simulink library "Lab_Library"  (R2022b)
settings: Solver=VariableStepAuto  StartTime=0.0  StopTime=10.0  RelTol=1e-3
undefined symbols (not defined in the file): IO397
libraries: slrealtimeiplib x7, slrealtimeseriallib x1, speedgoatlib_fpga_spi x1, speedgoatlib_fpga x1
settings Model: Creator=l-zirwin  LastModifiedBy=l-zirwin

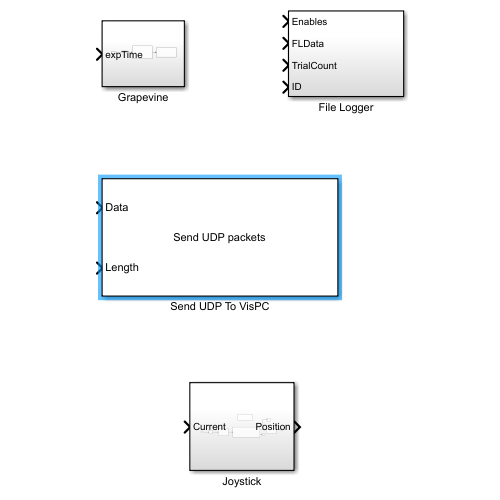
[thumbnail: Simulink's stored preview of the top-level diagram]
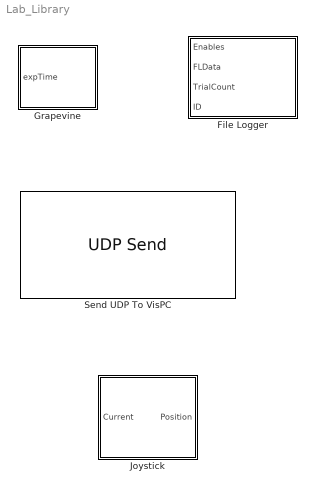
== system Lab_Library ==
  File Logger : Subsystem
  Grapevine : Subsystem
  Joystick : Subsystem
  Send UDP To VisPC : slrealtimeiplib/UDP Send  useHostTargetConn=off  toAddress='192.168.44.2'  toPort=11114  sampleTime=-1  enableMessage=off  ipAddress='192.168.44.1'  localPort=11114

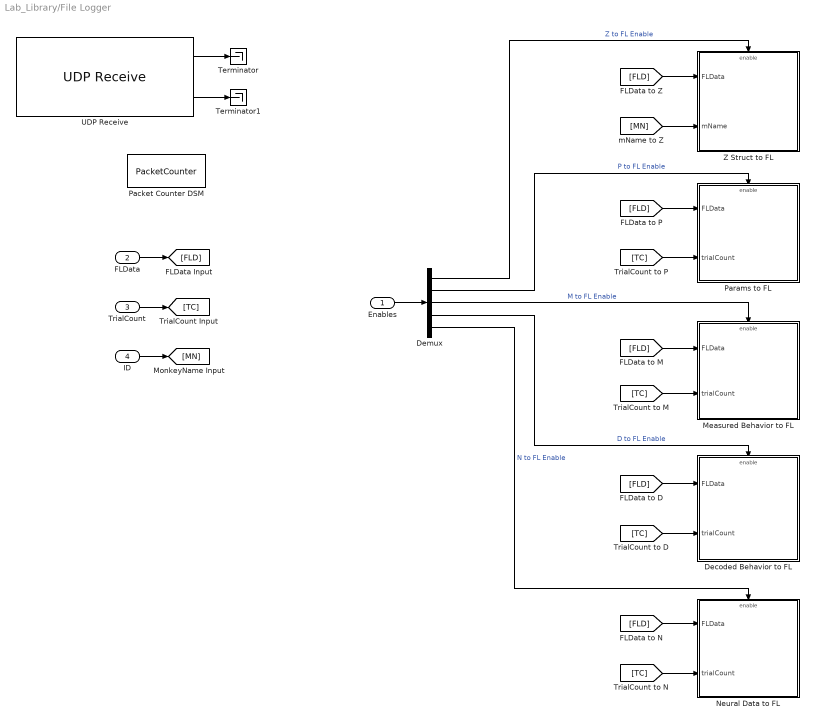
== system Lab_Library/File Logger ==
  Enables : Inport  OutDataTypeStr=uint8  PortDimensions=[1 5]
  FLData : Inport  Port=2  OutDataTypeStr=Bus: FileLoggerEntry
  TrialCount : Inport  Port=3
  ID : Inport  Port=4
  Decoded Behavior to FL : Subsystem
  Demux : Demux  Outputs=5
  Measured Behavior to FL : Subsystem
  Neural Data to FL : Subsystem
  Packet Counter DSM : DataStoreMemory  DataStoreName=PacketCounter  WriteAfterWriteMsg=warning  ShowAdditionalParam=off  OutDataTypeStr=uint32  Dimensions=1
  Params to FL : Subsystem
  Terminator : Terminator
  Terminator1 : Terminator
  UDP Receive : slrealtimeiplib/UDP Receive  useHostTargetConn=off  ipAddress='192.168.43.1'  localPort=11114  rcvWidth=16  rcvFmAny=off  fmAddress='192.168.43.2'  sampleTime=-1  enableMessage=off  maxPackets=1
  Z Struct to FL : Subsystem
  wires:
  TrialCount/1 -> [TC]
  FLData/1 -> [FLD]
  [FLD] -> Z Struct to FL/1(FLData)
  [FLD] -> Params to FL/1(FLData)
  [FLD] -> Measured Behavior to FL/1(FLData)
  [FLD] -> Decoded Behavior to FL/1(FLData)
  [FLD] -> Neural Data to FL/1(FLData)
  [TC] -> Params to FL/2(trialCount)
  [TC] -> Measured Behavior to FL/2(trialCount)
  [TC] -> Decoded Behavior to FL/2(trialCount)
  [TC] -> Neural Data to FL/2(trialCount)
  Enables/1 -> Demux/1
  Demux/3 -> Measured Behavior to FL/Enable  "M to FL Enable"
  Demux/4 -> Decoded Behavior to FL/Enable  "D to FL Enable"
  Demux/5 -> Neural Data to FL/Enable  "N to FL Enable"
  Demux/2 -> Params to FL/Enable  "P to FL Enable"
  Demux/1 -> Z Struct to FL/Enable  "Z to FL Enable"
  ID/1 -> [MN]
  [MN] -> Z Struct to FL/2(mName)
  UDP Receive/2 -> Terminator1/1
  UDP Receive/1 -> Terminator/1

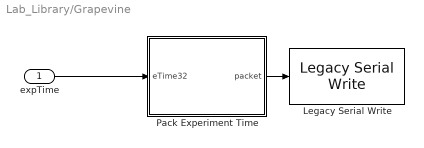
== system Lab_Library/Grapevine ==
  expTime : Inport
  Legacy Serial Write : slrealtimeseriallib/Mainboard/Legacy Serial Write  port=Legacy Serial Port 2  dtype=count+32 bit uint  sampletime=-1
  Pack Experiment Time : MATLAB Function  TreatAsAtomicUnit=on
  wires:
  expTime/1 -> Pack Experiment Time/1(eTime32)
  Pack Experiment Time/1(packet) -> Legacy Serial Write/1

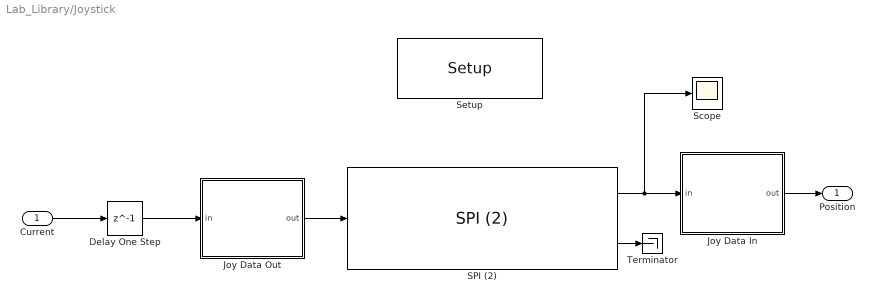
== system Lab_Library/Joystick ==
  Current : Inport
  Delay One Step : Delay  DelayLength=1
  Joy Data In : MATLAB Function  TreatAsAtomicUnit=on
  Joy Data Out : MATLAB Function  TreatAsAtomicUnit=on
  SPI (2) : speedgoatlib_fpga_spi/SPI (2)  id=1  chan=[1]  samp_time=.001  board=IO397-50k  pciSlot=-1  role=Master  sync_mode=off  multislave_mode=off  write_only=off  read_only=off  enableDma=off  multislave_chan=[1]  cpol=[0]  cpha=[0]  frequency=[1e6]  frequency_eff=1e6  delay_start=[2e-6]  delay_start_eff=2e-6  delay_interword=[1e-6]  delay_interword_eff=1e-6  delay_stop=[1e-6]  delay_stop_eff=1e-6  delay_compensation=[100e-9]  delay_compensation_eff=106.7e-9  words_per_frame=[2]  dynamic_words_per_frame=off  bits_per_word=[16]  bit_shift_lsb_first=[0]  no_cs=off  clock_timeout=[1e-6]  clock_timeout_eff=1E-06
      settings: SourceProductName=Simulink Real-Time: Speedgoat I/O Blockset
  Scope : Scope
  Setup : speedgoatlib_fpga/Setup/Setup  board=IO397-50k  id=1  device_id=1  frontIO=None  rearIO=None  bitstreamFile=speedgoat_IO397_50k_Comms.mat  rev=4.000000  timestamp_string=18/02/22 13:58:38  fpgaFreq=75 MHz  fpgaTick=13.33 ns  ProgSpiFlash=off  ProgBPIFlash=off  pciSlot=-1  PullRPort0=pull-up 3.3V  VioPort0=3.3V  PullRPort1=pull-up 3.3V  VioPort1=3.3V  PullRPort2=pull-up 3.3V  VioPort2=3.3V  PullRPort3=pull-up 3.3V  VioPort3=3.3V  PullRPort4=pull-up 3.3V  VioPort4=3.3V  PullRPort5=pull-up 3.3V  VioPort5=3.3V  PullRPort6=pull-up 3.3V  VioPort6=3.3V  diffLineTermination_rear1=on  diffLineTermination_rear2=on  diffLineTermination_rear3=on  diffLineTermination_rear4=on  diffLineTermination_rear5=on  diffLineTermination_rear6=on  diffLineTermination_rear7=on  diffLineTermination_rear8=on  PullRPort15=pull-up 3.3V  PullRPort31=pull-up 3.3V  PullRPort47=pull-up 3.3V  PullRPort63=pull-up 3.3V  diffLineTermination_1=on  diffLineTermination_2=on  diffLineTermination_3=on  diffLineTermination_4=on  diffLineTermination_5=on  diffLineTermination_6=on  diffLineTermination_7=on  diffLineTermination_8=on
      settings: SourceProductName=Simulink Real-Time: Speedgoat I/O Blockset
  Terminator : Terminator
  Position : Outport
  wires:
  Joy Data Out/1(out) -> SPI (2)/1
  SPI (2)/1 -> Scope/1, Joy Data In/1(in)
  Joy Data In/1(out) -> Position/1
  SPI (2)/2 -> Terminator/1
  Current/1 -> Delay One Step/1
  Delay One Step/1 -> Joy Data Out/1(in)

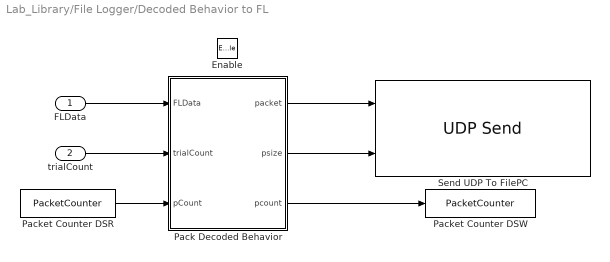
== system Lab_Library/File Logger/Decoded Behavior to FL ==
  FLData : Inport
  trialCount : Inport  Port=2
  Enable : EnablePort
  Pack Decoded Behavior : MATLAB Function  TreatAsAtomicUnit=on
  Packet Counter DSR : DataStoreRead  DataStoreName=PacketCounter  SampleTime=.001  IndexOptions=Index vector (dialog)  Indices=1  OutputSizes=1
  Packet Counter DSW : DataStoreWrite  DataStoreName=PacketCounter  IndexOptions=Index vector (dialog)  Indices=1  OutputSizes=1
  Send UDP To FilePC : slrealtimeiplib/UDP Send  useHostTargetConn=off  toAddress='192.168.43.2'  toPort=11114  sampleTime=-1  enableMessage=off  ipAddress='192.168.43.1'  localPort=11114
  wires:
  FLData/1 -> Pack Decoded Behavior/1(FLData)
  trialCount/1 -> Pack Decoded Behavior/2(trialCount)
  Packet Counter DSR/1 -> Pack Decoded Behavior/3(pCount)
  Pack Decoded Behavior/1(packet) -> Send UDP To FilePC/1
  Pack Decoded Behavior/3(pcount) -> Packet Counter DSW/1
  Pack Decoded Behavior/2(psize) -> Send UDP To FilePC/2

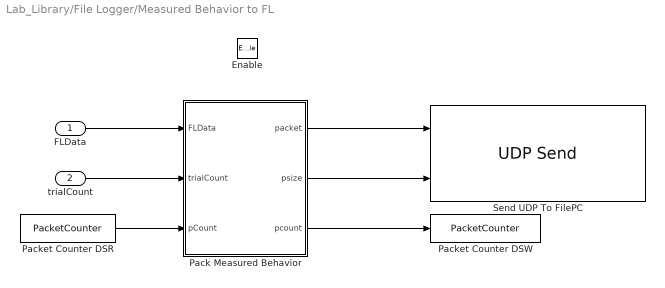
== system Lab_Library/File Logger/Measured Behavior to FL ==
  FLData : Inport
  trialCount : Inport  Port=2
  Enable : EnablePort
  Pack Measured Behavior : MATLAB Function  TreatAsAtomicUnit=on
  Packet Counter DSR : DataStoreRead  DataStoreName=PacketCounter  SampleTime=.001  IndexOptions=Index vector (dialog)  Indices=1  OutputSizes=1
  Packet Counter DSW : DataStoreWrite  DataStoreName=PacketCounter  IndexOptions=Index vector (dialog)  Indices=1  OutputSizes=1
  Send UDP To FilePC : slrealtimeiplib/UDP Send  useHostTargetConn=off  toAddress='192.168.43.2'  toPort=11114  sampleTime=-1  enableMessage=off  ipAddress='192.168.43.1'  localPort=11114
  wires:
  FLData/1 -> Pack Measured Behavior/1(FLData)
  trialCount/1 -> Pack Measured Behavior/2(trialCount)
  Packet Counter DSR/1 -> Pack Measured Behavior/3(pCount)
  Pack Measured Behavior/3(pcount) -> Packet Counter DSW/1
  Pack Measured Behavior/1(packet) -> Send UDP To FilePC/1
  Pack Measured Behavior/2(psize) -> Send UDP To FilePC/2

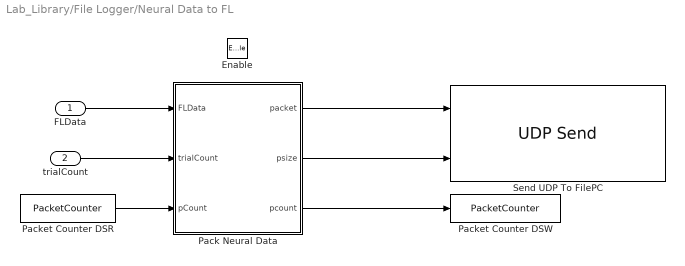
== system Lab_Library/File Logger/Neural Data to FL ==
  FLData : Inport
  trialCount : Inport  Port=2
  Enable : EnablePort
  Pack Neural Data : MATLAB Function  TreatAsAtomicUnit=on
  Packet Counter DSR : DataStoreRead  DataStoreName=PacketCounter  SampleTime=.001  IndexOptions=Index vector (dialog)  Indices=1  OutputSizes=1
  Packet Counter DSW : DataStoreWrite  DataStoreName=PacketCounter  IndexOptions=Index vector (dialog)  Indices=1  OutputSizes=1
  Send UDP To FilePC : slrealtimeiplib/UDP Send  useHostTargetConn=off  toAddress='192.168.43.2'  toPort=11114  sampleTime=-1  enableMessage=off  ipAddress='192.168.43.1'  localPort=11114
  wires:
  FLData/1 -> Pack Neural Data/1(FLData)
  trialCount/1 -> Pack Neural Data/2(trialCount)
  Packet Counter DSR/1 -> Pack Neural Data/3(pCount)
  Pack Neural Data/3(pcount) -> Packet Counter DSW/1
  Pack Neural Data/1(packet) -> Send UDP To FilePC/1
  Pack Neural Data/2(psize) -> Send UDP To FilePC/2

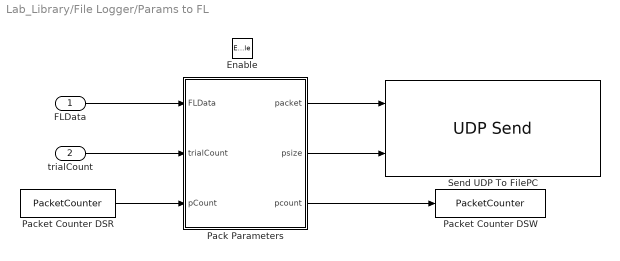
== system Lab_Library/File Logger/Params to FL ==
  FLData : Inport
  trialCount : Inport  Port=2
  Enable : EnablePort
  Pack Parameters : MATLAB Function  TreatAsAtomicUnit=on
  Packet Counter DSR : DataStoreRead  DataStoreName=PacketCounter  SampleTime=.001  IndexOptions=Index vector (dialog)  Indices=1  OutputSizes=1
  Packet Counter DSW : DataStoreWrite  DataStoreName=PacketCounter  IndexOptions=Index vector (dialog)  Indices=1  OutputSizes=1
  Send UDP To FilePC : slrealtimeiplib/UDP Send  useHostTargetConn=off  toAddress='192.168.43.2'  toPort=11114  sampleTime=-1  enableMessage=off  ipAddress='192.168.43.1'  localPort=11114
  wires:
  FLData/1 -> Pack Parameters/1(FLData)
  trialCount/1 -> Pack Parameters/2(trialCount)
  Packet Counter DSR/1 -> Pack Parameters/3(pCount)
  Pack Parameters/1(packet) -> Send UDP To FilePC/1
  Pack Parameters/2(psize) -> Send UDP To FilePC/2
  Pack Parameters/3(pcount) -> Packet Counter DSW/1

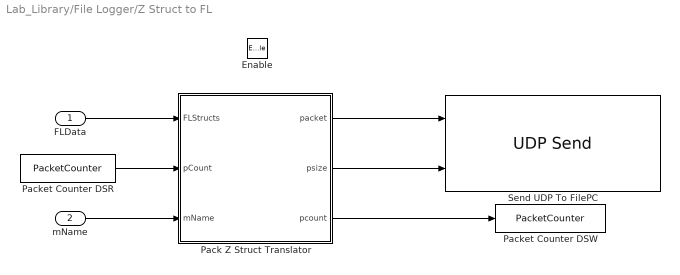
== system Lab_Library/File Logger/Z Struct to FL ==
  FLData : Inport
  mName : Inport  Port=2
  Enable : EnablePort
  Pack Z Struct Translator : MATLAB Function  TreatAsAtomicUnit=on
  Packet Counter DSR : DataStoreRead  DataStoreName=PacketCounter  SampleTime=.001  IndexOptions=Index vector (dialog)  Indices=1  OutputSizes=1
  Packet Counter DSW : DataStoreWrite  DataStoreName=PacketCounter  IndexOptions=Index vector (dialog)  Indices=1  OutputSizes=1
  Send UDP To FilePC : slrealtimeiplib/UDP Send  useHostTargetConn=off  toAddress='192.168.43.2'  toPort=11114  sampleTime=-1  enableMessage=off  ipAddress='192.168.43.1'  localPort=11114
  wires:
  FLData/1 -> Pack Z Struct Translator/1(FLStructs)
  Packet Counter DSR/1 -> Pack Z Struct Translator/2(pCount)
  mName/1 -> Pack Z Struct Translator/3(mName)
  Pack Z Struct Translator/3(pcount) -> Packet Counter DSW/1
  Pack Z Struct Translator/1(packet) -> Send UDP To FilePC/1
  Pack Z Struct Translator/2(psize) -> Send UDP To FilePC/2

== matlab function Lab_Library/Grapevine/Pack Experiment Time ==
  data: eTime32 input uint32 size=1; packet output uint32 size=[1,5]
function packet = TypecastETime(eTime32)

packet = uint32([4, typecast(eTime32, 'uint8')]);

== matlab function Lab_Library/Joystick/Joy Data Out ==
  data: in input single size=1; out output uint32 size=[1,2]
function out = FormatJoyDataOut(in)

out = uint32(typecast(single(in), 'uint16'));

== matlab function Lab_Library/Joystick/Joy Data In ==
  data: in input uint32 size=[1,2]; out output uint16 size=[1,2]
function out = FormatJoyDataIn(in)

in = single(in);

xmin = 1.142e4;
xmax = 1.507e4;
ymin = 2.006e3;
ymax = 4.949e3;

x = single((in(1) - xmin)/(xmax - xmin));
y = single((in(2) - ymin)/(ymax - ymin));

if (x < 0)
    x = single(0);
elseif (x > 1)
    x = single(1);
end

if (y < 0)
    y = single(0);
elseif (y > 1)
    y = single(1);
end

out = uint16([x,y].*[1600, 900]);

%  out = uint16(([x, y]/5).*[1600,900]);

== matlab function Lab_Library/File Logger/Z Struct to FL/Pack Z Struct Translator ==
  data: packet output uint8 size=[1,1500]; FLStructs input Bus: FileLoggerEntry; pCount input uint32 size=1; psize output double size=1; mName input uint8; pcount output uint32 size=1
% This translates the FileLoggerEntry struct array to a Z struct description
% string for the Z Struct Translator script to use at a later date.
%
% FL Packet:[packetCount(4b), packetType(1b), data(xb)]
%   -> First 2 bytes of non-ZPacket data are the trialCount
%
% Z Struct descriptor: 'fieldname1-datatype1-numElements1-fieldname2-...'
%
%   Written by Zach Irwin for the Chestek Lab, 2012
%%%%%%%%%%%%%%%%%%%%%%%%%%%%%%%%%%%%%%%%%%%%%%%%%%%%%%%%%%%%%%%%%%%%%%%%%%%

function [packet, psize, pcount] = genZPacket(FLStructs, pCount, mName)
%#codegen

sb = uint8('-'); % Spacer byte
headers = uint8([':P:'; ':M:'; ':D:'; ':N:']); % File Type headers

%Current packet size (with headers/monkey name, max size = 1500 bytes):
psize = double(4 + 1 + length(mName) + 1);

%Initialize packet (packetCount, packetType, mNameSize, mName, padding):
packet = uint8([typecast(uint32(pCount), 'uint8'), uint8(0), uint8(length(mName)), mName',zeros(1,1500-psize)]);

%Sort FLStructs into FileTypes (Params, mBehavior, dBehavior, Neural):
idxs = zeros(5,length(FLStructs));

for i = 1:length(FLStructs)

     switch FLStructs(i).FileType
         case 2 % Measured Behavior File Type
             idxs(2, nnz(idxs(2,:)) + 1) = i;
         case 3 % Decoded Behavior File Type
             idxs(3, nnz(idxs(3,:)) + 1) = i;
         case 4 % Neural Data File Type
             idxs(4, nnz(idxs(4,:)) + 1) = i;
         case 5 % Trial Begin Parameter File Type
             idxs(1, nnz(idxs(1,:)) + 1) = i;
         case 6 % Trial End Parameter File Type
             idxs(5, nnz(idxs(1,:)) + 1) = i;
     end
    
end

%Iterate through each File Type, add data to packet:
for i = 1:4
    
    % Collect structs for the current File Type:
    nidxs = idxs(i, :); % Current set of indices for ith File Type
    
    if (i == 1)
        nidxs5 = idxs(5,:); % Indices for the End Parameters File Type
        data = [FLStructs(nidxs(nidxs~=0)), FLStructs(nidxs5(nidxs5~=0))];
    else
        data = FLStructs(nidxs(nidxs ~= 0)); % Current File Type Structs
    end
    
    % Add correct File Type header:
    start = psize + uint16(1); stop = psize + uint16(3);
    packet(start:stop) = headers(i,:);
    
    % Update number of elements in the packet:
    psize = psize + double(3);
    
    % Iterate through the File Type structs & add to packet:
    for j = 1:length(data)
        
        % Recover non-NULL fieldName string:
        fname = data(j).FieldName(data(j).FieldName ~= 0);
        
        % Recover non-NULL dataType string:
        dtype = data(j).DataType(data(j).DataType ~= 0);
        
        % If either of these is empty, generate an error:
        if (isempty(fname) || isempty(dtype))
            error('An FLStruct FieldName or DataType is NULL. Don''t include extraneous FLStructs.');
        end
        
        % Recover numElements byte:
        numel = data(j).NumElements;
        
        % Size of all of these elements + 3 spacer bytes:
        inum = length(fname) + length(dtype) + length(numel) + 3;
        
        % Pack this set of bytes into the packet:
        start = psize + uint16(1); stop = psize + uint16(inum);
        packet(start:stop) = uint8([fname, sb, dtype, sb, numel, sb]);
        
        % Update number of elements in the packet:
        psize = psize + double(inum);
        
    end
    
end

% Update packet count:
pcount = pCount + uint32(1);

end

== matlab function Lab_Library/File Logger/Params to FL/Pack Parameters ==
  data: FLData input Bus: FileLoggerEntry; packet output uint8 size=[1,1500]; trialCount input uint16 size=1; pCount input uint32 size=1; psize output size=1; pcount output uint32 size=1
% This packs a vector of the trial parameters to send to the File Logger
%
% FL Packet:[runTime(4b), packetType(1b), data(xb)]
%   -> First 2 bytes of non-ZPacket data are the trialCount
%
%   Written by Zach Irwin for the Chestek Lab, 2012
%%%%%%%%%%%%%%%%%%%%%%%%%%%%%%%%%%%%%%%%%%%%%%%%%%%%%%%%%%%%%%%%%%%%%%%%%%%

function [packet, psize, pcount] = genPPacket(FLData, trialCount, pCount)
%#codegen

persistent prev_count

%This function gets called twice per trial, prev_count lets us know which
%type of trial parameters to send (FileType 5 or FileType 6)
if (isempty(prev_count))
    prev_count = -1;        
end

%Figure out which FileType to send:
if (prev_count == trialCount)
    ftype = 6;  %Send the Trial Wrap-up parameters
else
    ftype = 5;  %Send Trial Begin parameters
    prev_count = double(trialCount); %Reset count
end

%Convert runTime & trialCount to uint8 vectors:
rt = typecast(uint32(pCount), 'uint8');
tc = typecast(uint16(trialCount), 'uint8');

%Initialize packet vector [runTime(x4), packetType(x1), trialCount(x2), data(x1493)]:
packet = uint8([rt, uint8(ftype), tc, zeros(1,1493)]);

%Keep track of no. of bytes in the packet:
psize = double(7); %4 runTime bytes, 1 packetType byte, and 2 trialCount bytes

for i = 1:length(FLData)
    
    %Skip FLData structs without parameter data (fileType = 5 or 6):
   if (FLData(i).FileType ~= ftype)
       continue;
   end
   
   %Get non-zero data from struct:
   ddata = FLData(i).Data(1:FLData(i).NumElements); %Elements as doubles
   
   %Cast data to correct type, then uint8s for packing:
   type = char(FLData(i).DataType(FLData(i).DataType ~= 0));
   if (strcmp(type, 'uint8'))
       data = uint8(ddata);
   elseif (strcmp(type, 'int8'))
       data = typecast(int8(ddata),'uint8');
   elseif (strcmp(type, 'uint16'))
       data = typecast(uint16(ddata),'uint8');
   elseif (strcmp(type, 'int16'))
       data = typecast(int16(ddata),'uint8');
   elseif (strcmp(type, 'uint32'))
       data = typecast(uint32(ddata),'uint8');
   elseif (strcmp(type, 'int32'))
       data = typecast(int32(ddata),'uint8');
   elseif (strcmp(type, 'single'))
       data = typecast(single(ddata),'uint8');
   elseif (strcmp(type, 'double'))
       data = typecast(ddata,'uint8');
   else
       data = uint8(0); % Should never happen
   end
   
   %Add data to packet:
   start = psize + uint16(1); stop = psize + uint16(length(data));
   packet(start:stop) = data;
   
   %Update number of elements in the packet:
   psize = psize + double(length(data));
   
   if (psize > 1500)
       error('Packet size reached: P Packet type');
   end
   
end

%Update packet count:
pcount = pCount + uint32(1);
end

== matlab function Lab_Library/File Logger/Measured Behavior to FL/Pack Measured Behavior ==
  data: FLData input Bus: FileLoggerEntry; packet output uint8 size=[1,1500]; trialCount input uint16 size=1; pCount input uint32 size=1; psize output size=1; pcount output uint32 size=1
% This packs a vector of the measured behavior to send to the File Logger
%
% FL Packet:[runTime(4b), packetType(1b), data(xb)]
%   -> First 2 bytes of non-ZPacket data are the trialCount
%
%   Written by Zach Irwin for the Chestek Lab, 2012
%%%%%%%%%%%%%%%%%%%%%%%%%%%%%%%%%%%%%%%%%%%%%%%%%%%%%%%%%%%%%%%%%%%%%%%%%%%

function [packet, psize, pcount] = genMPacket(FLData, trialCount, pCount)
%#codegen

%Convert runTime & trialCount to uint8 vectors:
rt = typecast(uint32(pCount), 'uint8');
tc = typecast(uint16(trialCount), 'uint8');

%Initialize packet vector [runTime(x4), packetType(x1), trialCount(x2), data(x1493)]:
packet = uint8([rt, uint8(2), tc, zeros(1,1493)]);

%Keep track of no. of bytes in the packet:
psize = double(7); %4 runTime bytes, 1 packetType byte, and 2 trialCount bytes

for i = 1:length(FLData)
    
    %Skip FLData strucuts without meas. behavior data (fileType = 2):
   if (FLData(i).FileType ~= 2)
       continue;
   end
   
   %Get non-zero data from struct:
   ddata = FLData(i).Data(1:FLData(i).NumElements); %Elements as doubles
   
   %Cast data to correct type, then uint8s for packing:
   type = char(FLData(i).DataType(FLData(i).DataType ~= 0));
   if (strcmp(type, 'uint8'))
       data = uint8(ddata);
   elseif (strcmp(type, 'int8'))
       data = typecast(int8(ddata),'uint8');
   elseif (strcmp(type, 'uint16'))
       data = typecast(uint16(ddata),'uint8');
   elseif (strcmp(type, 'int16'))
       data = typecast(int16(ddata),'uint8');
   elseif (strcmp(type, 'uint32'))
       data = typecast(uint32(ddata),'uint8');
   elseif (strcmp(type, 'int32'))
       data = typecast(int32(ddata),'uint8');
   elseif (strcmp(type, 'single'))
       data = typecast(single(ddata),'uint8');
   elseif (strcmp(type, 'double'))
       data = typecast(ddata,'uint8');
   else
       data = uint8(0); % Should never happen
   end
   
   %Add data to packet:
   start = psize + uint16(1); stop = psize + uint16(length(data));
   packet(start:stop) = data;
   
   %Update number of elements in the packet:
   psize = psize + double(length(data));
   
   if (psize > 1500)
       error('Packet size reached: M Packet type');
   end
   
end

%Update packet count:
pcount = pCount + uint32(1);
end

== matlab function Lab_Library/File Logger/Decoded Behavior to FL/Pack Decoded Behavior ==
  data: FLData input Bus: FileLoggerEntry; packet output uint8 size=[1,1500]; trialCount input uint16 size=1; pCount input uint32 size=1; psize output size=1; pcount output uint32 size=1
% This packs a vector of the decoded behavior to send to the File Logger
%
% FL Packet:[runTime(4b), packetType(1b), data(xb)]
%   -> First 2 bytes of non-ZPacket data are the trialCount
%
%   Written by Zach Irwin for the Chestek Lab, 2012
%%%%%%%%%%%%%%%%%%%%%%%%%%%%%%%%%%%%%%%%%%%%%%%%%%%%%%%%%%%%%%%%%%%%%%%%%%%

function [packet, psize, pcount] = genDPacket(FLData, trialCount, pCount)
%#codegen

%Convert runTime & trialCount to uint8 vectors:
rt = typecast(uint32(pCount), 'uint8');
tc = typecast(uint16(trialCount), 'uint8');

%Initialize packet vector [runTime(x4), packetType(x1), trialCount(x2), data(x1493)]:
packet = uint8([rt, uint8(3), tc, zeros(1,1493)]);

%Keep track of no. of bytes in the packet:
psize = double(7); %4 runTime bytes, 1 packetType byte, and 2 trialCount bytes

for i = 1:length(FLData)
    
    %Skip FLData strucuts without dec. behavior data (fileType = 3):
   if (FLData(i).FileType ~= 3)
       continue;
   end
   
   %Get non-zero data from struct:
   ddata = FLData(i).Data(1:FLData(i).NumElements); %Elements as doubles
   
   %Cast data to correct type, then uint8s for packing:
   type = char(FLData(i).DataType(FLData(i).DataType ~= 0));
   if (strcmp(type, 'uint8'))
       data = uint8(ddata);
   elseif (strcmp(type, 'int8'))
       data = typecast(int8(ddata),'uint8');
   elseif (strcmp(type, 'uint16'))
       data = typecast(uint16(ddata),'uint8');
   elseif (strcmp(type, 'int16'))
       data = typecast(int16(ddata),'uint8');
   elseif (strcmp(type, 'uint32'))
       data = typecast(uint32(ddata),'uint8');
   elseif (strcmp(type, 'int32'))
       data = typecast(int32(ddata),'uint8');
   elseif (strcmp(type, 'single'))
       data = typecast(single(ddata),'uint8');
   elseif (strcmp(type, 'double'))
       data = typecast(ddata,'uint8');
   else
       data = uint8(0); % Should never happen
   end
   
   %Add data to packet:
   start = psize + uint16(1); stop = psize + uint16(length(data));
   packet(start:stop) = data;
   
   %Update number of elements in the packet:
   psize = psize + double(length(data));
   
   if (psize > 1500)
       error('Packet size reached: D Packet type');
   end
   
end

%Update packet count:
pcount = pCount + uint32(1);
end

== matlab function Lab_Library/File Logger/Neural Data to FL/Pack Neural Data ==
  data: FLData input Bus: FileLoggerEntry; packet output uint8 size=[1,1500]; trialCount input uint16 size=1; pCount input uint32 size=1; psize output size=1; pcount output uint32 size=1
    % This packs a vector of the Neural data to send to the File Logger
%
% FL Packet:[runTime(4b), packetType(1b), data(xb)]
%   -> First 2 bytes of non-ZPacket data are the trialCount
%
% *NOTE: Neural packets have an "end packet" character(255) as the last
% byte in the packet. This is to support variable length spike channels.
%
%   Written by Zach Irwin for the Chestek Lab, 2012
%%%%%%%%%%%%%%%%%%%%%%%%%%%%%%%%%%%%%%%%%%%%%%%%%%%%%%%%%%%%%%%%%%%%%%%%%%%

function [packet, psize, pcount] = genNPacket(FLData, trialCount, pCount)
%#codegen

%Convert runTime & trialCount to uint8 vectors:
rt = typecast(uint32(pCount), 'uint8');
tc = typecast(uint16(trialCount), 'uint8');

%Initialize packet vector [runTime(x4), packetType(x1), trialCount(x2), data(x1493)]:
packet = uint8([rt, uint8(4), tc, zeros(1,1493)]);

%Keep track of no. of bytes in the packet:
psize = double(7); %4 runTime bytes, 1 packetType byte, and 2 trialCount bytes

for i = 1:length(FLData)
    
    %Skip FLData structs without neural data (fileType = 4):
   if (FLData(i).FileType ~= 4)
       continue;
   end
   
   %Get non-zero data from struct:
   if (FLData(i).NumElements == 0)
        ddata = FLData(i).Data(FLData(i).Data ~= 0); %Elements as doubles
   else
        ddata = FLData(i).Data(1:FLData(i).NumElements); %Elements as doubles
   end
   
   %Cast data to correct type, then uint8s for packing:
   type = char(FLData(i).DataType(FLData(i).DataType ~= 0));
   if (strcmp(type, 'uint8'))
       data = uint8(ddata);
   elseif (strcmp(type, 'int8'))
       data = typecast(int8(ddata),'uint8');
   elseif (strcmp(type, 'uint16'))
       data = typecast(uint16(ddata),'uint8');
   elseif (strcmp(type, 'int16'))
       data = typecast(int16(ddata),'uint8');
   elseif (strcmp(type, 'uint32'))
       data = typecast(uint32(ddata),'uint8');
   elseif (strcmp(type, 'int32'))
       data = typecast(int32(ddata),'uint8');
   elseif (strcmp(type, 'single'))
       data = typecast(single(ddata),'uint8');
   elseif (strcmp(type, 'double'))
       data = typecast(ddata,'uint8');
   else
       data = uint8(0); % Should never happen
   end
   
   %Add data to packet:
   start = psize + uint16(1); stop = psize + uint16(length(data));
   packet(start:stop) = data;
   
   %Update number of elements in the packet:
   psize = psize + double(length(data));
   
   if (psize >= 1500)
       error('Packet size reached: N Packet type');
   end
   
end

%Add End Packet byte:
packet(psize+uint16(1)) = uint8(255);
psize = psize + double(1);

%Update packet count:
pcount = pCount + uint32(1);

end
